simulink model "gm_GEN_LRCLK"  (R2023b)
settings: Solver=FixedStepAuto  StartTime=0.0  StopTime=10.0  RelTol=1e-3
undefined symbols (not defined in the file or in its folder): cnt1_LRCLK
libraries: hdlsllib x1
settings Model: Creator=31651  LastModifiedBy=31651
settings OptimizationCC: BlockReduction=off  ConditionallyExecuteInputs=off  DefaultParameterBehavior=Inlined
settings DebuggingCC: AlgebraicLoopMsg=error  InheritedTsInSrcMsg=none
settings HardwareCC: ProdBitPerPointer=32  ProdBitPerSizeT=32  ProdBitPerPtrDiffT=32  ProdLargestAtomicFloat=None  ProdIntDivRoundTo=Undefined  ProdEndianess=Unspecified  ProdWordSize=32  ProdHWDeviceType=ASIC/FPGA->ASIC/FPGA  TargetBitPerPointer=64  TargetBitPerSizeT=64  TargetBitPerPtrDiffT=64  TargetLongLongMode=on  TargetIntDivRoundTo=Zero  TargetEndianess=LittleEndian  TargetWordSize=64  TargetHWDeviceType=Custom Processor->MATLAB Host Computer  ProdEqTarget=off

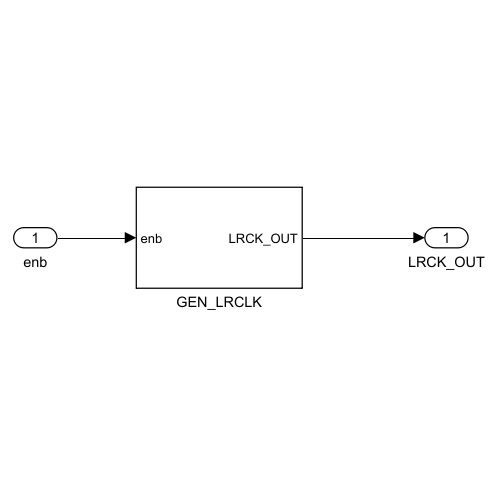
[thumbnail: Simulink's stored preview of the top-level diagram]
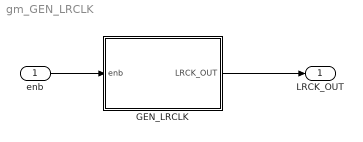
== system gm_GEN_LRCLK ==
  enb : Inport  OutDataTypeStr=boolean  PortDimensions=1  SampleTime=0.2
  GEN_LRCLK : Subsystem
  LRCK_OUT : Outport  SampleTime=0.2  VectorParamsAs1DForOutWhenUnconnected=off
  wires:
  enb/1 -> GEN_LRCLK/1(enb)
  GEN_LRCLK/1(LRCK_OUT) -> LRCK_OUT/1

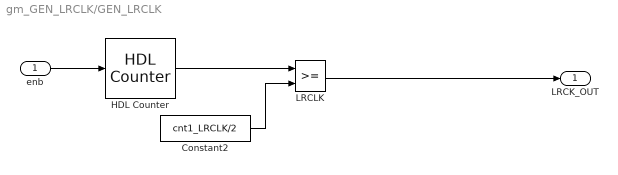
== system gm_GEN_LRCLK/GEN_LRCLK ==
  enb : Inport  OutDataTypeStr=boolean  PortDimensions=1  SampleTime=0.2
  Constant2 : Constant  Value=cnt1_LRCLK/2  OutDataTypeStr=uint16
  HDL Counter : hdlsllib/Sources/HDL Counter  CountType=Count limited  CountInit=0  CountStep=1  CountMax=cnt1_LRCLK  CountFromType=Initial value  CountFrom=0  CountResetPort=off  CountLoadPort=off  CountEnbPort=on  CountDirPort=off  CountHitOutputPort=off  CountDataType=Unsigned  CountWordLen=16  CountFracLen=0  CountSampTime=1
  LRCLK : RelationalOperator  OutDataTypeStr=boolean  InputSameDT=off
  LRCK_OUT : Outport  OutDataTypeStr=boolean  SampleTime=0.2
  wires:
  enb/1 -> HDL Counter/1
  Constant2/1 -> LRCLK/2
  HDL Counter/1 -> LRCLK/1
  LRCLK/1 -> LRCK_OUT/1
